simulink model "mpp_tracker"  (R2023b)
settings: Solver=VariableStepAuto  StartTime=0.0  StopTime=Tsim  RelTol=1e-3
model workspace (MAT data in the model file):
  Ts = 0.001
  Tsim = 1
undefined symbols (not defined in the file): DiscIntNeverNeededParam
libraries: slpidlib x1
settings Model: Creator=alex8  LastModifiedBy=alex8

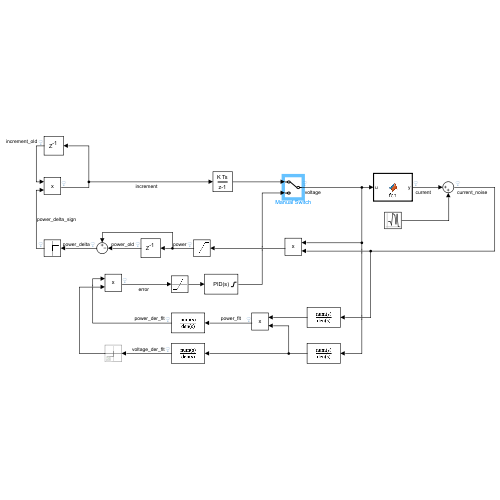
[thumbnail: Simulink's stored preview of the top-level diagram]
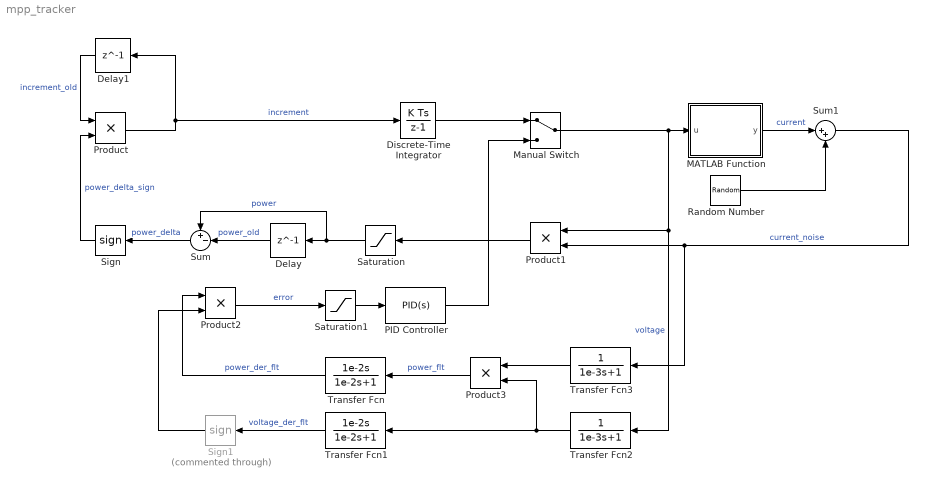
== system mpp_tracker ==
  Delay : Delay  DelayLength=1  SampleTime=Ts
  Delay1 : Delay  DelayLength=1  InitialCondition=10e-3  SampleTime=Ts
  Discrete-Time Integrator : DiscreteIntegrator  gainval=1/Ts  InitialCondition=0.1  SampleTime=Ts  ICPrevOutput=DiscIntNeverNeededParam  ICPrevScaledInput=DiscIntNeverNeededParam
  MATLAB Function : MATLAB Function  TreatAsAtomicUnit=on
  Manual Switch : ManualSwitch
  PID Controller : slpidlib/PID Controller  Controller=PID  Form=Parallel  TimeDomain=Continuous-time  UseExternalTs=off  SampleTime=-1  IntegratorMethod=Forward Euler  FilterMethod=Forward Euler  ControllerParametersSource=internal  P=0.3  I=1e3  UseKiTs=off  D=0  N=100  UseFilter=on  TunerSelectOption=Transfer Function Based (PID Tuner App)  InitialConditionSource=internal  InitialConditionForIntegrator=0.3  InitialConditionForFilter=0  DifferentiatorICPrevScaledInput=0  ExternalReset=none  TrackingMode=off  Kt=1  LimitOutput=on  SatLimitsSource=internal  UpperSaturationLimit=0.65  LowerSaturationLimit=0  LinearizeAsGain=on  AntiWindupMode=clamping  Kb=1  LimitIntegrator=off  UpperIntegratorSaturationLimit=inf  LowerIntegratorSaturationLimit=-inf  POutMin=[]  POutMax=[]  IOutMin=[]  IOutMax=[]  DOutMin=[]  DOutMax=[]  NOutMin=[]  NOutMax=[]  SumOutMin=[]  SumOutMax=[]  SaturationOutMin=[]  SaturationOutMax=[]  PParamMin=[]  PParamMax=[]  IParamMin=[]  IParamMax=[]  DParamMin=[]  DParamMax=[]  NParamMin=[]  NParamMax=[]  KbParamMin=[]  KbParamMax=[]  KtParamMin=[]  KtParamMax=[]  KbOutMin=[]  KbOutMax=[]  KtOutMin=[]  KtOutMax=[]  IntegratorOutMin=[]  IntegratorOutMax=[]  FilterOutMin=[]  FilterOutMax=[]  SumI1OutMin=[]  SumI1OutMax=[]  SumI2OutMin=[]  SumI2OutMax=[]  SumI3OutMin=[]  SumI3OutMax=[]  SumI4OutMin=[]  SumI4OutMax=[]  SumDOutMin=[]  SumDOutMax=[]  DifferentiatorOutMin=[]  DifferentiatorOutMax=[]  FilterDiffOutCoefMin=[]  FilterDiffOutCoefMax=[]  ReciprocalOutMin=[]  ReciprocalOutMax=[]  SumDenOutMin=[]  SumDenOutMax=[]  SumNumOutMin=[]  SumNumOutMax=[]  DivideOutMin=[]  DivideOutMax=[]  UdiffTsProdOutMin=[]  UdiffTsProdOutMax=[]  NTsProdOutMin=[]  NTsProdOutMax=[]  UintegralTsProdOutMin=[]  UintegralTsProdOutMax=[]  UngainTsProdOutMin=[]  UngainTsProdOutMax=[]  ClampingZeroOutDataTypeStr=Inherit: Inherit via back propagation  ClampingZeroOutMin=[]  ClampingZeroOutMax=[]  FilterDenConstantOutDataTypeStr=Inherit: Inherit via back propagation  FilterDenConstantOutMin=[]  FilterDenConstantOutMax=[]  PCopyOutDataTypeStr=Inherit: Inherit via back propagation  PCopyOutMin=[]  PCopyOutMax=[]  NCopyOutDataTypeStr=Inherit: Inherit via back propagation  NCopyOutMin=[]  NCopyOutMax=[]  IntegratorContinuousStateAttributes=''  IntegratorStateMustResolveToSignalObject=off  IntegratorRTWStateStorageClass=Auto  FilterContinuousStateAttributes=''  FilterStateMustResolveToSignalObject=off  FilterRTWStateStorageClass=Auto  ParallelPVariant=InternalParameters  IdealPVariant=Disabled  IVariant=InternalParameters  DVariant=InternalParameters  IntegratorVariant=Continuous  SatVariant=Enabled  AWVariant=ContClampingParallel  PCopyVariant=Disabled  TRVariant=Disabled  FdbkBlocksVariant=Forward  IdealPFdbkVariant=Disabled  SatFdbkVariant=Disabled  DerivativeFilterVariant=ContFilter  NVariant=InternalParameters  NCopyVariant=Disabled  FilterICVariant=InternalICsFilter  IntegratorICVariant=InternalICs  ExternalResetVariant=Disabled  TRSumVariant=Passthrough  SumFdbkVariant=Disabled  SumVariant=Sum_PID  TsampFilterVariant=InternalTs  TsampNgainVariant=Passthrough  TsampIntegralVariant=Disabled_SignalSpec  ExternalSaturationOutDataTypeStr=Inherit: Same as second input
  Product{,1..3} (4 alike) : Product
  Random Number : RandomNumber  Variance=0.001  SampleTime=Ts/10
  Saturation : Saturate  UpperLimit=Inf  LowerLimit=1e-3
  Saturation1 : Saturate  UpperLimit=10e-3
  Sign : Signum
  Sign1 : Signum  Commented=through
  Sum : Sum  Inputs=+-|
  Sum1 : Sum  Inputs=|++
  Transfer Fcn : TransferFcn  Numerator=[1e-2 0]  Denominator=[1e-2 1]
  Transfer Fcn1 : TransferFcn  Numerator=[1e-2 0]  Denominator=[1e-2 1]
  Transfer Fcn2 : TransferFcn  Denominator=[1e-3 1]
  Transfer Fcn3 : TransferFcn  Denominator=[1e-3 1]
  wires:
  Manual Switch/1 -> Transfer Fcn2/1, Product1/1, MATLAB Function/1(u)  "voltage"
  Product/1 -> Delay1/1, Discrete-Time Integrator/1  "increment"
  Delay/1 -> Sum/2  "power_old"
  Product1/1 -> Saturation/1
  Sign/1 -> Product/2  "power_delta_sign"
  Sum1/1 -> Transfer Fcn3/1, Product1/2  "current_noise"
  Sum/1 -> Sign/1  "power_delta"
  Saturation/1 -> Delay/1, Sum/1  "power"
  Delay1/1 -> Product/1  "increment_old"
  MATLAB Function/1(y) -> Sum1/1  "current"
  Random Number/1 -> Sum1/2
  Transfer Fcn/1 -> Product2/1  "power_der_flt"
  Discrete-Time Integrator/1 -> Manual Switch/1
  Transfer Fcn1/1 -> Sign1/1  "voltage_der_flt"
  Product2/1 -> Saturation1/1  "error"
  Transfer Fcn2/1 -> Product3/2, Transfer Fcn1/1
  Product3/1 -> Transfer Fcn/1  "power_flt"
  Transfer Fcn3/1 -> Product3/1
  PID Controller/1 -> Manual Switch/2
  Sign1/1 -> Product2/2
  Saturation1/1 -> PID Controller/1

== matlab function mpp_tracker/MATLAB Function ==
  data: u input; y output; par_fit parameter
function y = fcn(u, par_fit)

y = fcell_expl(u, par_fit);
